simulink model "force_control"  (R2025a)
settings: Solver=FixedStepDiscrete  StartTime=0.0  StopTime=inf  FixedStep=0.01  RelTol=1e-3  EnableMultiTasking=on
PreLoadFcn:
  | frs = FrankaRobotSettings;
undefined symbols (not defined in the file): DiscIntNeverNeededParam
libraries: simulink x1, franka_simulink x1
settings Model: ExtModeTrigDuration=10000  Creator=vasi_ko  LastModifiedBy=kvasios
settings SolverCC: AlgebraicLoopSolver=TrustRegion
settings DataIOCC: LimitDataPoints=on  SaveFormat=Array  ReturnWorkspaceOutputs=off
settings OptimizationCC: EnhancedBackFolding=on  PassReuseOutputArgsThreshold=0.0  OptimizeBlockOrder=speed  DifferentSizesBufferReuse=on  OptimizationCustomize=off
settings DebuggingCC: SolverPrmCheckMsg=warning  ParameterTunabilityLossMsg=error  UnconnectedInputMsg=warning  UnconnectedOutputMsg=warning  UnconnectedLineMsg=warning  SFUnexpectedBacktrackingDiag=warning  SFNoUnconditionalDefaultTransitionDiag=warning  SFExecutionAtInitializationDiag=none  ArithmeticOperatorsInVariantConditions=warning
settings HardwareCC: ProdBitPerLong=64.0  ProdHWDeviceType=Intel->x86-64 (Linux 64)
settings ModelReferenceCC: EnableRefExpFcnMdlSchedulingChecks=on  PropagateSignalLabelsOutOfModel=off
settings SFSimCC: SimUseLocalCustomCode=off  MATLABDynamicMemAlloc=off  CustomCodeUndefinedFunction=UseInterfaceOnly  SimTargetLang=C++  SimDLTargetLibrary=mkl-dnn
settings RTWCC: HardwareBoard=Generic Linux AMD64 Board  RTWVerbose=off  RTWUseLocalCustomCode=off  BuildConfiguration=Faster Runs  TargetLang=C++  GPUComputeCapability=3.5  DLArmComputeVersion=19.05
settings CodeAppCC: ForceParamTrailComments=on  OperatorAnnotations=on
settings GRTTargetCC: ExtMode=on  ExtModeStaticAlloc=on  ExtModeMexFile=ext_xcp  ExtModeIntrfLevel=Level2 - Open  TargetLangStandard=C++14 (ISO)
settings ConfigComp: CovMetricSettings=dw  CovSaveCumulativeToWorkspaceVar=on  CovSaveSingleToWorkspaceVar=on  CovExternalEMLEnable=off  CovSFcnEnable=off

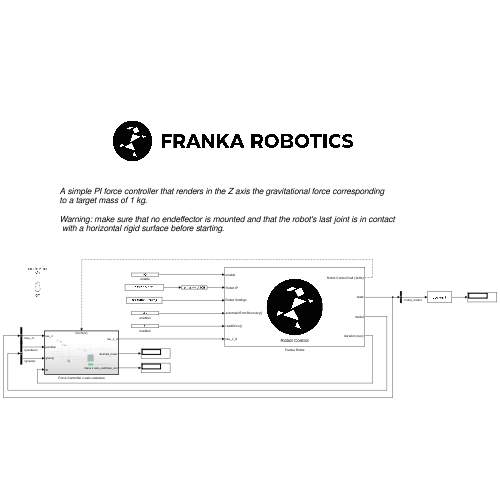
[thumbnail: Simulink's stored preview of the top-level diagram]
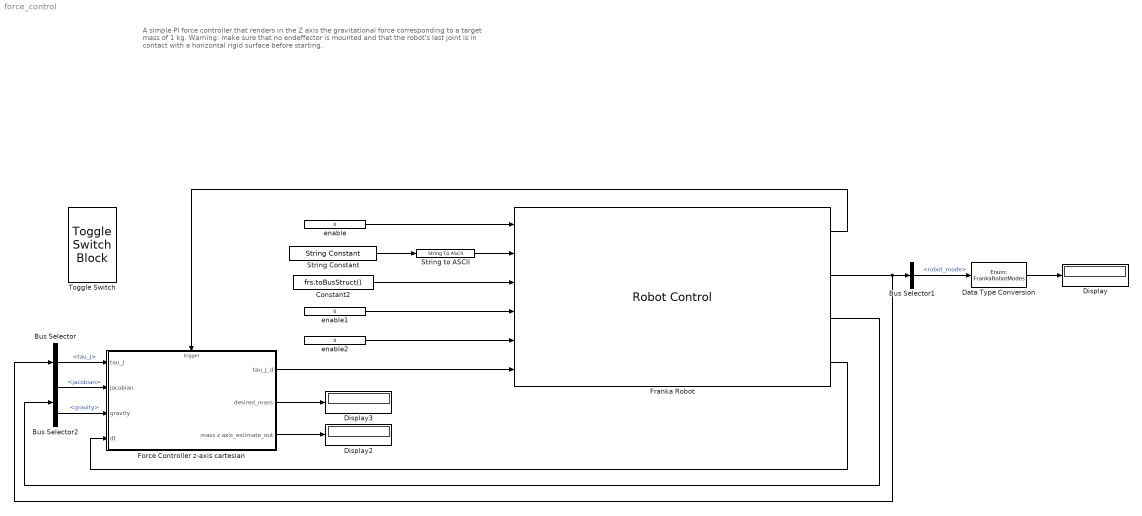
== system force_control ==
  note: A simple PI force controller that renders in the Z axis the gravitational force corresponding
      | to a target mass of 1 kg.
      |
      | Warning: make sure that no endeffector is mounted and that the robot's last joint is in contact
      |  with a horizontal rigid surface before starting.
  Bus Selector : BusSelector  OutputSignals=tau_J
  Bus Selector1 : BusSelector  OutputSignals=robot_mode
  Bus Selector2 : BusSelector  OutputSignals=jacobian,gravity
  Constant2 : Constant  Value=frs.toBusStruct()  OutDataTypeStr=Bus: FrankaRobotSettingsBus
  Data Type Conversion : DataTypeConversion  OutDataTypeStr=Enum: FrankaRobotModes  SaturateOnIntegerOverflow=off  RndMeth=Floor
  Display : Display
  Display2 : Display
  Display3 : Display
  Force Controller z-axis cartesian : Subsystem
      settings: RTWSystemCode=Nonreusable function
  Franka Robot : franka_simulink/Robot Control  control_mode=Torques
      settings: SourceProductName=Franka Robotics Simulink Support Package
  String Constant : StringConstant  String="\"172.16.0.2\""
  String to ASCII : StringToASCII  OutputVectorSize=16
  Toggle Switch : ToggleSwitchBlock
  enable : Constant  Value=0  SampleTime=-1
  enable1 : Constant  Value=0  SampleTime=-1
  enable2 : Constant  Value=0  SampleTime=-1
  wires:
  Constant2/1 -> Franka Robot/3
  enable2/1 -> Franka Robot/5
  String to ASCII/1 -> Franka Robot/2
  Franka Robot/1 -> Force Controller z-axis cartesian/Trigger
  Franka Robot/2 -> Bus Selector1/1, Bus Selector/1
  enable1/1 -> Franka Robot/4
  String Constant/1 -> String to ASCII/1
  Franka Robot/4 -> Force Controller z-axis cartesian/4(dt)
  Bus Selector1/1 -> Data Type Conversion/1  "<robot_mode>"
  Franka Robot/3 -> Bus Selector2/1
  Bus Selector/1 -> Force Controller z-axis cartesian/1(tau_J)  "<tau_J>"
  Data Type Conversion/1 -> Display/1
  Bus Selector2/1 -> Force Controller z-axis cartesian/2(jacobian)  "<jacobian>"
  Bus Selector2/2 -> Force Controller z-axis cartesian/3(gravity)  "<gravity>"
  Force Controller z-axis cartesian/3(mass z axis_estimate_out) -> Display2/1
  Force Controller z-axis cartesian/2(desired_mass) -> Display3/1
  Force Controller z-axis cartesian/1(tau_J_d) -> Franka Robot/6
  enable/1 -> Franka Robot/1

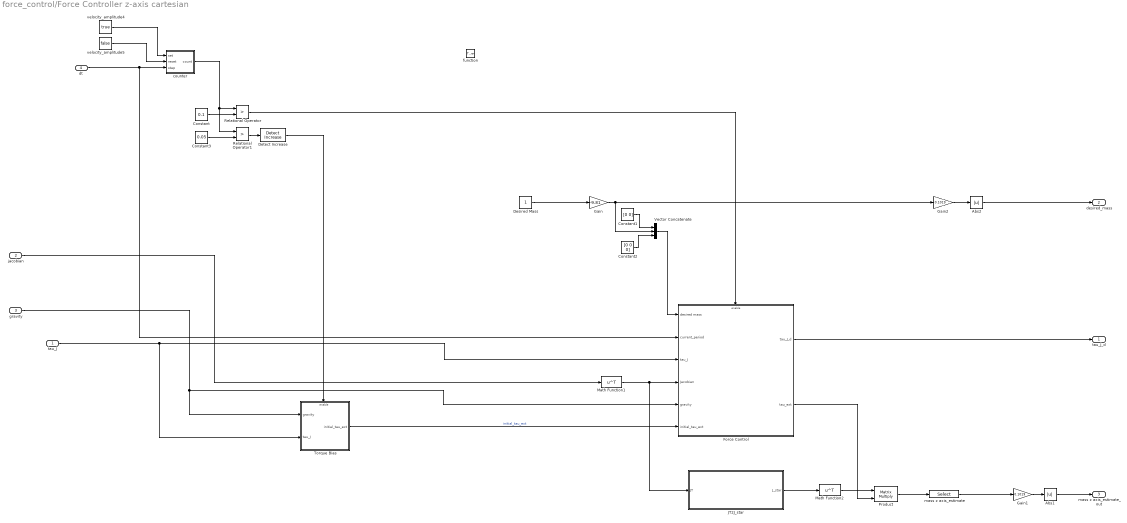
== system force_control/Force Controller z-axis cartesian ==
  tau_J : Inport
  jacobian : Inport  Port=2
  gravity : Inport  Port=3
  dt : Inport  Port=4
  function : TriggerPort  TriggerType=function-call  VariantControl=(inherit)
  Abs1 : Abs  SaturateOnIntegerOverflow=off
  Abs2 : Abs  SaturateOnIntegerOverflow=off
  Constant : Constant  Value=0.1
  Constant1 : Constant  Value=[0 0]
  Constant2 : Constant  Value=[0 0 0]
  Constant3 : Constant  Value=0.05
  Desired Mass : Constant
  Detect Increase : simulink/Logic and Bit Operations/Detect Increase  vinit=0.0  OutDataTypeStr=boolean
  Force Control : Subsystem
  Gain : Gain  Gain=-9.81
  Gain1 : Gain  Gain=0.1019
  Gain2 : Gain  Gain=0.1019
  JT2J_star : MATLAB Function  TreatAsAtomicUnit=on
  Math Function1 : Math  Operator=transpose  SignedPower=on
  Math Function2 : Math  Operator=transpose  SignedPower=on
  Product : Product  Multiplication=Matrix(*)
  Relational Operator : RelationalOperator  Operator=>  OutDataTypeStr=boolean  InputSameDT=off
  Relational Operator1 : RelationalOperator  Operator=>  OutDataTypeStr=boolean  InputSameDT=off
  Torque Bias : Subsystem
  Vector Concatenate : Concatenate  NumInputs=3
  counter : Subsystem
  mass z axis_estimate : Selector  InputPortWidth=6  IndexOptions=Index vector (dialog)  Indices=3  OutputSizes=1
  velocity_amplitude4 : Constant  Value=true  VectorParams1D=off
  velocity_amplitude5 : Constant  Value=false  VectorParams1D=off
  tau_J_d : Outport  VectorParamsAs1DForOutWhenUnconnected=off
  desired_mass : Outport  Port=2  VectorParamsAs1DForOutWhenUnconnected=off
  mass z axis_estimate_out : Outport  Port=3  VectorParamsAs1DForOutWhenUnconnected=off
  wires:
  Constant/1 -> Relational Operator/2
  Constant1/1 -> Vector Concatenate/1
  Abs1/1 -> mass z axis_estimate_out/1
  Gain2/1 -> Abs2/1
  Constant3/1 -> Relational Operator1/2
  Abs2/1 -> desired_mass/1
  jacobian/1 -> Math Function1/1
  Force Control/1(tau_J_d) -> tau_J_d/1
  Gain/1 -> Gain2/1, Vector Concatenate/2
  Constant2/1 -> Vector Concatenate/3
  Product/1 -> mass z axis_estimate/1
  Torque Bias/1(initial_tau_ext) -> Force Control/6(initial_tau_ext)  "initial_tau_ext"
  Detect Increase/1 -> Torque Bias/Enable
  Vector Concatenate/1 -> Force Control/1(desired mass)
  Desired Mass/1 -> Gain/1
  counter/1(count) -> Relational Operator/1, Relational Operator1/1
  Math Function2/1 -> Product/1
  Relational Operator/1 -> Force Control/Enable
  JT2J_star/1(J_star) -> Math Function2/1
  Gain1/1 -> Abs1/1
  Relational Operator1/1 -> Detect Increase/1
  Force Control/2(tau_ext) -> Product/2
  Math Function1/1 -> JT2J_star/1(JT), Force Control/4(Jacobian)
  tau_J/1 -> Force Control/3(tau_J), Torque Bias/2(tau_J)
  mass z axis_estimate/1 -> Gain1/1
  gravity/1 -> Torque Bias/1(gravity), Force Control/5(gravity)
  velocity_amplitude5/1 -> counter/2(reset)
  dt/1 -> Force Control/2(current_period), counter/3(step)
  velocity_amplitude4/1 -> counter/1(set)

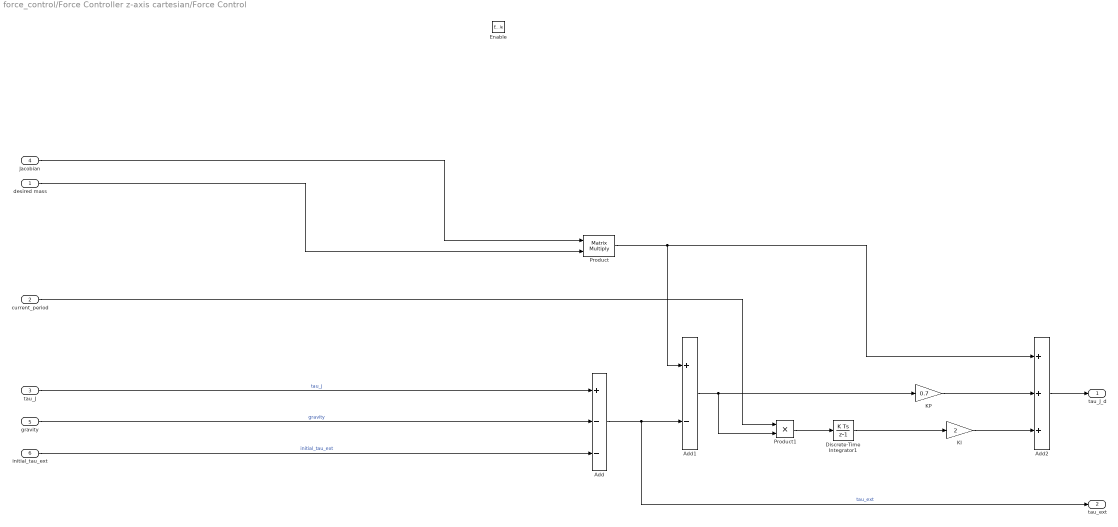
== system force_control/Force Controller z-axis cartesian/Force Control ==
  desired mass : Inport
  current_period : Inport  Port=2
  tau_J : Inport  Port=3
  Jacobian : Inport  Port=4
  gravity : Inport  Port=5
  initial_tau_ext : Inport  Port=6
  Enable : EnablePort
  Add : Sum  Inputs=+--
  Add1 : Sum  Inputs=+-
  Add2 : Sum  Inputs=+++
  Discrete-Time Integrator1 : DiscreteIntegrator  SampleTime=-1  ICPrevOutput=DiscIntNeverNeededParam  ICPrevScaledInput=DiscIntNeverNeededParam
  KI : Gain  Gain=2
  KP : Gain  Gain=0.7
  Product : Product  Multiplication=Matrix(*)
  Product1 : Product
  tau_J_d : Outport  InitialOutput=zeros(7,1)  VectorParamsAs1DForOutWhenUnconnected=off
  tau_ext : Outport  Port=2  InitialOutput=zeros(7,1)  VectorParamsAs1DForOutWhenUnconnected=off
  wires:
  Jacobian/1 -> Product/1
  tau_J/1 -> Add/1  "tau_J"
  gravity/1 -> Add/2  "gravity"
  Add/1 -> tau_ext/1, Add1/2  "tau_ext"
  Add1/1 -> Product1/2, KP/1
  Add2/1 -> tau_J_d/1
  Product1/1 -> Discrete-Time Integrator1/1
  current_period/1 -> Product1/1
  KI/1 -> Add2/3
  initial_tau_ext/1 -> Add/3  "initial_tau_ext"
  Product/1 -> Add1/1, Add2/1
  KP/1 -> Add2/2
  desired mass/1 -> Product/2
  Discrete-Time Integrator1/1 -> KI/1

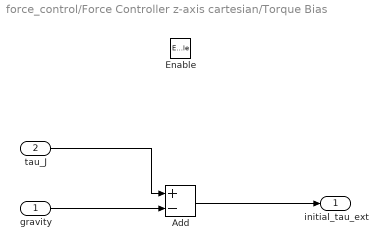
== system force_control/Force Controller z-axis cartesian/Torque Bias ==
  gravity : Inport
  tau_J : Inport  Port=2
  Enable : EnablePort
  Add : Sum  Inputs=+-
  initial_tau_ext : Outport  InitialOutput=zeros(7,1)  VectorParamsAs1DForOutWhenUnconnected=off
  wires:
  tau_J/1 -> Add/1
  gravity/1 -> Add/2
  Add/1 -> initial_tau_ext/1

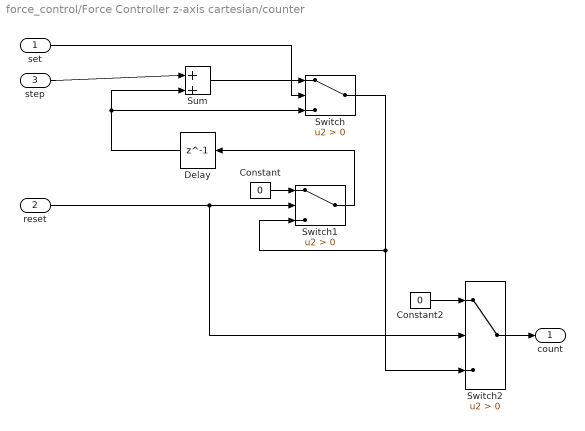
== system force_control/Force Controller z-axis cartesian/counter ==
  set : Inport  OutDataTypeStr=boolean
  reset : Inport  Port=2  OutDataTypeStr=boolean
  step : Inport  Port=3  OutDataTypeStr=double
  Constant : Constant  Value=0  OutDataTypeStr=double
  Constant2 : Constant  Value=0  OutDataTypeStr=double
  Delay : Delay  DelayLength=1  InitialCondition=0
  Sum : Sum  Inputs=|++
  Switch : Switch  Criteria=u2 > Threshold  SaturateOnIntegerOverflow=off  InputSameDT=off
  Switch1 : Switch  Criteria=u2 > Threshold  OutDataTypeStr=double  SaturateOnIntegerOverflow=off  InputSameDT=off
  Switch2 : Switch  Criteria=u2 > Threshold  OutDataTypeStr=double  SaturateOnIntegerOverflow=off  InputSameDT=off
  count : Outport  OutDataTypeStr=double  VectorParamsAs1DForOutWhenUnconnected=off
  wires:
  Switch2/1 -> count/1
  Constant2/1 -> Switch2/1
  Sum/1 -> Switch/1
  set/1 -> Switch/2
  Switch/1 -> Switch1/3, Switch2/3
  step/1 -> Sum/1
  Delay/1 -> Sum/2, Switch/3
  reset/1 -> Switch1/2, Switch2/2
  Constant/1 -> Switch1/1
  Switch1/1 -> Delay/1

== matlab function force_control/Force Controller z-axis cartesian/JT2J_star ==
  data: JT input; J_star output
function J_star = JT2J_star(JT)
%#codegen

J = JT';
% low isotropic damping, the value should be much smaller than lambda_max^2
beta =0;
% damping added in singular directions, we chose it to be equal to
% threshold
% lambda_max = singularity_threshold_inverse_kinematics; 
% SVD decomposition
[U,S,~] = svd(J);
sigma = diag(S);
% rank
singularity_threshold_inverse_kinematics = eps;
r = sum(sigma > singularity_threshold_inverse_kinematics);
% initilizing damping
  lambda_square_vector = zeros(6,1);
if r==6 % damping in full rank case is zero
    lambda_square_vector = zeros(6,1);
else % daamping in rank deficient cases
%     sigma_singular = sigma(r+1:6);
%     lambda_square_vector(r+1:6) = ...
%         (1 - (sigma_singular/ singularity_threshold_inverse_kinematics).^2) *...
%         lambda_max^2;
end
J_star =  JT * U * diag(1./(sigma.^2+lambda_square_vector+beta^2*ones(6,1)))*U';

end
